simulink model "lb552_usrp_tx_am_fdm"  (R2018b)
settings: Solver=VariableStepAuto  StartTime=0.0  StopTime=inf  RelTol=1e-3
undefined symbols (not defined in the file): fdesignblkfcn, gcbh
libraries: dspvision x3, dspfdesign x3, dsparch4 x2, dspsrcs4 x2, dspmlti4 x2, commsdrhw_v2 x1
settings Model: SimulationMode=accelerator  Creator=Григорий Фокин  LastModifiedBy=Григорий Фокин
settings SFSimCC: SimUseLocalCustomCode=off
settings RTWCC: RTWUseLocalCustomCode=off
settings CodeAppCC: StateflowObjectComments=on

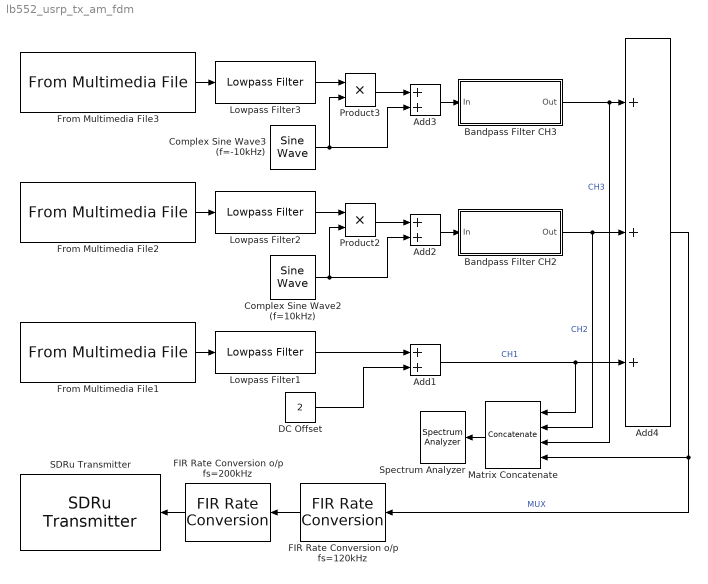
== system lb552_usrp_tx_am_fdm ==
  Add1 : Sum
  Add2 : Sum
  Add3 : Sum
  Add4 : Sum  Inputs=+++
  Bandpass Filter CH2 : Subsystem  DialogController=fdesignblkfcn  InitFcn=fdesignblkfcn(gcbh, {'InitFcn'});  mask(Bandpass Filter){}
      mask help: Design a bandpass filter
      settings: CopyFcn=fdesignblkfcn(gcbh, {'CopyFcn'});
      mask Help: helpview(mapfilelocation('dsp'), 'dspbandpassfilter');
      mask Display: disp('Bandpass');
  Bandpass Filter CH3 : Subsystem  DialogController=fdesignblkfcn  InitFcn=fdesignblkfcn(gcbh, {'InitFcn'});  mask(Bandpass Filter){}
      mask help: Design a bandpass filter
      settings: CopyFcn=fdesignblkfcn(gcbh, {'CopyFcn'});
      mask Help: helpview(mapfilelocation('dsp'), 'dspbandpassfilter');
      mask Display: disp('Bandpass');
  Complex Sine Wave2 (f=10kHz) : dspsrcs4/Sine Wave  Amplitude=2  Frequency=10e3  Phase=0  SampleMode=Discrete  OutComplex=Complex  CompMethod=Trigonometric fcn  TableSize=Speed  SampleTime=1/48e3  SamplesPerFrame=600  ResetState=Restart at time zero  OutputFrames=off  dataType=double  wordLen=16  udDataType=sfix(16)  fracBitsMode=Best precision  numFracBits=15  OutDataTypeStr=double  LastOutDataTypeStr=double
  Complex Sine Wave3 (f=-10kHz) : dspsrcs4/Sine Wave  Amplitude=2  Frequency=-10e3  Phase=0  SampleMode=Discrete  OutComplex=Complex  CompMethod=Trigonometric fcn  TableSize=Speed  SampleTime=1/48e3  SamplesPerFrame=600  ResetState=Restart at time zero  OutputFrames=off  dataType=double  wordLen=16  udDataType=sfix(16)  fracBitsMode=Best precision  numFracBits=15  OutDataTypeStr=double  LastOutDataTypeStr=double
  DC Offset : Constant  Value=2
  FIR Rate Conversion o/p fs=120kHz : dspmlti4/FIR Rate Conversion  FilterSource=Dialog parameters  L=5  h=firpm(100, [0 16000 24000 240e3/2]/(240e3/2), [1 1 0 0], [1 1],20)  M=2  FilterObject=FRC  roundingMode=Floor  overflowMode=off  firstCoeffDataTypeStr=Inherit: Same word length as input  firstCoeffMin=[]  firstCoeffMax=[]  firstCoeffLastDataTypeStr=Inherit: Same word length as input  outputDataTypeStr=Inherit: Same as accumulator  outputMin=[]  outputMax=[]  outputLastDataTypeStr=Inherit: Same as accumulator
      settings: SourceProductName=DSP System Toolbox  SourceProductBaseCode=DS
  FIR Rate Conversion o/p fs=200kHz : dspmlti4/FIR Rate Conversion  FilterSource=Dialog parameters  L=5  h=firpm(100, [0 16e3 24e3 600e3/2]/(600e3/2), [1 1 0 0], [1 1],20)  M=3  FilterObject=FRC  roundingMode=Floor  overflowMode=off  firstCoeffDataTypeStr=Inherit: Same word length as input  firstCoeffMin=[]  firstCoeffMax=[]  firstCoeffLastDataTypeStr=Inherit: Same word length as input  outputDataTypeStr=Inherit: Same as accumulator  outputMin=[]  outputMax=[]  outputLastDataTypeStr=Inherit: Same as accumulator
      settings: SourceProductName=DSP System Toolbox  SourceProductBaseCode=DS
  From Multimedia File1 : dspvision/From Multimedia File  inputFilename=C:\Users\Григорий Фокин\Documents\MATLAB\sut_study\dcsdr\audio_sources\music1_mono48kHz.wav  loop=on  numPlays=inf  outputStreams=Audio only  videoDataType=single  audioDataType=single  inheritSampleTime=on  userDefinedSampleTime=1/30  noAudioOutput=off  isIntensityVideo=off  fourcc=RGB  colorVideoFormat=Separate color signals  outputEOF=off  dataOrg=Column-major  audioFrameSize=600  computeAudioFrameSize=off  outSamplingMode=Sample based
      settings: SourceProductBaseCode=VP
  From Multimedia File2 : dspvision/From Multimedia File  inputFilename=C:\Users\Григорий Фокин\Documents\MATLAB\sut_study\dcsdr\audio_sources\music2_mono48kHz.wav  loop=on  numPlays=inf  outputStreams=Audio only  videoDataType=single  audioDataType=single  inheritSampleTime=on  userDefinedSampleTime=1/30  noAudioOutput=off  isIntensityVideo=off  fourcc=RGB  colorVideoFormat=Separate color signals  outputEOF=off  dataOrg=Column-major  audioFrameSize=600  computeAudioFrameSize=off  outSamplingMode=Sample based
      settings: SourceProductBaseCode=VP
  From Multimedia File3 : dspvision/From Multimedia File  inputFilename=C:\Users\Григорий Фокин\Documents\MATLAB\sut_study\dcsdr\audio_sources\music3_mono48kHz.wav  loop=on  numPlays=inf  outputStreams=Audio only  videoDataType=single  audioDataType=single  inheritSampleTime=on  userDefinedSampleTime=1/30  noAudioOutput=off  isIntensityVideo=off  fourcc=RGB  colorVideoFormat=Separate color signals  outputEOF=off  dataOrg=Column-major  audioFrameSize=600  computeAudioFrameSize=off  outSamplingMode=Sample based
      settings: SourceProductBaseCode=VP
  Lowpass Filter1 : dspfdesign/Lowpass Filter  FilterType=IIR  DesignForMinimumOrder=on  FilterOrder=50  PassbandFrequency=4e3  StopbandFrequency=4.5e3  PassbandRipple=1  StopbandAttenuation=100  InheritSampleRate=off  SampleRate=48e3  SimulateUsing=Interpreted execution  roundingMode=Floor  coeffsDataTypeStr=fixdt(1,16)
  Lowpass Filter2 : dspfdesign/Lowpass Filter  FilterType=IIR  DesignForMinimumOrder=on  FilterOrder=50  PassbandFrequency=4e3  StopbandFrequency=4.5e3  PassbandRipple=1  StopbandAttenuation=100  InheritSampleRate=off  SampleRate=48e3  SimulateUsing=Interpreted execution  roundingMode=Floor  coeffsDataTypeStr=fixdt(1,16)
  Lowpass Filter3 : dspfdesign/Lowpass Filter  FilterType=IIR  DesignForMinimumOrder=on  FilterOrder=50  PassbandFrequency=4e3  StopbandFrequency=4.5e3  PassbandRipple=1  StopbandAttenuation=100  InheritSampleRate=off  SampleRate=48e3  SimulateUsing=Interpreted execution  roundingMode=Floor  coeffsDataTypeStr=fixdt(1,16)
  Matrix Concatenate : Concatenate  NumInputs=4  Mode=Multidimensional array  ConcatenateDimension=2
  Product2 : Product
  Product3 : Product
  SDRu Transmitter : commsdrhw_v2/SDRu Transmitter  rxtx=tx  initializeIPAddress=0  devMap=0  USRP2_IP=192.168.10.2  USRP_IP_X300=192.168.10.2  USRP_IP_X310=192.168.10.2  USRP_serialNumB210=F4E642  platform=B210  prevPlatform=B210  lastIPAddressPopup=192.168.10.2  USRP_ID=F4E642  LastIPAddress=192.168.10.2  ChannelMapping=1  centerFrequencySrc=Dialog  centerFrequency=1200e6  loOffsetSrc=Dialog  loOffset=0  gainSrc=Dialog  gain=70  PPSSource=Internal  clockSource=Internal  masterClkRateParam=6000000  masterClkRateB200=32e6  masterClkRateB210=6e6  masterClkRateX300=200e6  masterClkRateX310=200e6  decimInterpSrc=Dialog  decimInterp=30  USRP2_IP_NUM=[70 52 69 54 52 50]  frameLength=362  TransportDataType=int16  outputDatatype=Same as transport data type  overrunUnderrunPort=off  sampleTime=1  dboardInfo=|  HOST_DATA_PORT=30000  HOST_CONTROL_PORT=30001  USRP2_DATA_PORT=32769  USRP2_CONTROL_PORT=32768  bufferMode=Continuous streaming  EnableBurstMode=off  NumFramesInBurst=100
      | dbid: 0
      |           dbName: 'no db found'
      |          freqMin: 0
      |          freqMax: 0
      |          gainMin: 0
      |          gainMax: 0
      |     gainStepSize: 0
      settings: SourceProductName=Communications System Toolbox Support Package for USRP(R) Radio  SourceProductBaseCode=USRP
  Spectrum Analyzer : SpectrumAnalyzer
  wires:
  From Multimedia File3/1 -> Lowpass Filter3/1
  Lowpass Filter3/1 -> Product3/1
  Complex Sine Wave3 (f=-10kHz)/1 -> Product3/2, Add3/2
  Product3/1 -> Add3/1
  Add3/1 -> Bandpass Filter CH3/1(In)
  From Multimedia File2/1 -> Lowpass Filter2/1
  Lowpass Filter2/1 -> Product2/1
  Complex Sine Wave2 (f=10kHz)/1 -> Add2/2, Product2/2
  Product2/1 -> Add2/1
  Add2/1 -> Bandpass Filter CH2/1(In)
  From Multimedia File1/1 -> Lowpass Filter1/1
  Lowpass Filter1/1 -> Add1/1
  DC Offset/1 -> Add1/2
  Bandpass Filter CH3/1(Out) -> Matrix Concatenate/3, Add4/1  "CH3"
  Bandpass Filter CH2/1(Out) -> Matrix Concatenate/2, Add4/2  "CH2"
  Add1/1 -> Matrix Concatenate/1, Add4/3  "CH1"
  FIR Rate Conversion o/p fs=120kHz/1 -> FIR Rate Conversion o/p fs=200kHz/1
  FIR Rate Conversion o/p fs=200kHz/1 -> SDRu Transmitter/1
  Matrix Concatenate/1 -> Spectrum Analyzer/1
  Add4/1 -> FIR Rate Conversion o/p fs=120kHz/1, Matrix Concatenate/4  "MUX"

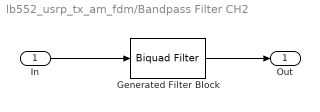
== system lb552_usrp_tx_am_fdm/Bandpass Filter CH2 ==
  In : Inport
  Generated Filter Block : dsparch4/Biquad Filter  Tag=BlockMethodSubSystem  FilterSource=Dialog parameters  CoeffSource=Specify via dialog  FilterObject=BQF  IIRFiltStruct=Direct form II  BiQuadCoeffs=[0.038316192503796788 0 -0.038316192503796788 1 -1.4647964271306377 0.94471193100608075;0.079066094669843379 0 -0.079066094669843379 1 -1.4478872277903894 0.92340777287438669;1.4987829140143871 0 -1.4987829140143871 1 -1.3806603018180272 0.84224281947975999;1.4262911444791184 0 -1.4262911444791184 1 0.58822635838518211 0.83492615482033494;0.12651868683152681 0 -0.12651868683152681 1 0.55132638249904897 0.75583004259253672;0.16278534730934865 0 -0.16278534730934865 1 -1.296689747244494 0.74843901978838578;0.17165110687366125 0 -0.17165110687366125 1 -1.2286258519522211 0.67826050546120453;1.2698273089041143 0 -1.2698273089041143 1 -1.2113783161788545 0.66128071032184788;0.20679428223229829 0 -0.20679428223229829 1 0.4575548300258192 0.59529881813215724;0.24203724548995642 0 -0.24203724548995642 1 -1.1410250658492758 0.59529322698110076;0.25085765032621515 0 -0.25085765032621515 1 -1.0676878443588245 0.53197037847147421;1.1262797117495502 0 -1.1262797117495502 1 -1.0487453100276105 0.51650173917589015;0.28689353541085916 0 -0.28689353541085916 1 0.3519417533947492 0.46218165129526773;0.32503837865502017 0 -0.32503837865502017 1 -0.96986311471358411 0.45593385510682483;1.0469924746795094 0 -1.0469924746795094 1 -0.88468241094327438 0.39740220475460397;0.36600529716476427 0 -0.36600529716476427 1 0.28503939659387562 0.39655389906045346;0.97025355161809479 0 -0.97025355161809479 1 -0.79108046931960629 0.34121276752547192;0.41170205075459598 0 -0.41170205075459598 1 0.21209573444104962 0.3380538505151206;0.89433754435568313 0 -0.89433754435568313 1 -0.68658006847610931 0.2885056716671846;0.81944502214295323 0 -0.81944502214295323 1 0.13161626710115215 0.28686560436176467;0.4635643277972038 0 -0.4635643277972038 1 0.041622402952489035 0.2438446895809836;0.74310982737617481 0 -0.74310982737617481 1 -0.56911862362598775 0.24200449865234008;0.52401642408429749 0 -0.52401642408429749 1 -0.060257140448974483 0.21085064512665316;0.6663474706877075 0 -0.6663474706877075 1 -0.439506581423658 0.20676604963866127;0.59171836614561801 0 -0.59171836614561801 1 -0.17601055769180582 0.1911208065583376;0.62712191993186295 0 -0.62712191993186295 1 -0.30478008617749719 0.18891158557670057;0.69966742183885922 0 -0.69966742183885922 1 -0.23904135382384317 0.18757452699095306;0.55330559254524614 0 -0.55330559254524614 1 -0.11634228576068456 0.19906897851393124;0.76917074247525774 0 -0.76917074247525774 1 -0.37209094308052626 0.19536146214396241;0.48617499002437708 0 -0.48617499002437708 1 -0.0076804609149881825 0.22592720694312463;0.83504112081969528 0 -0.83504112081969528 1 -0.50556036680048511 0.22257689527031324;0.42757746379429307 0 -0.42757746379429307 1 0.087951306871739937 0.26424643599944636;0.37860716298259545 0 -0.37860716298259545 1 -0.62953035756411801 0.2642209496329555;0.85794319827651577 0 -0.85794319827651577 1 -0.74034910133001519 0.31430206283391671;0.3156782373193644 0 -0.3156782373193644 1 0.17290986841503653 0.31151116853219307;0.72504748895787396 0 -0.72504748895787396 1 -0.83908419359333897 0.36896989749244613;0.68432655624176897 0 -0.68432655624176897 1 0.24940543484309963 0.36641429161510974;0.31152694401361014 0 -0.31152694401361014 1 0.31916944212687137 0.42846811137787677;0.68648839199988387 0 -0.68648839199988387 1 -0.92818196779966999 0.42640778321597184;0.30752809817970622 0 -0.30752809817970622 1 0.38347969139959992 0.49774535746443088;0.27169501816632724 0 -0.27169501816632724 1 -1.0099766818316462 0.48596263367743714;0.77277817453089304 0 -0.77277817453089304 1 -1.1048021701758253 0.56332975000387475;0.73508031520027628 0 -0.73508031520027628 1 0.42869230070154496 0.55473049811770636;0.29418562251053465 0 -0.29418562251053465 1 0.48546564941124593 0.6380818919747604;0.23621087503198085 0 -0.23621087503198085 1 -1.1765054758560753 0.62792026806225043;0.92057985047504121 0 -0.92057985047504121 1 -1.26281575076854 0.71287380301019321;0.19821400336650982 0 -0.19821400336650982 1 0.52563846635605715 0.70676158328244532 ...(+4917 chars)]  ScaleValues=[0.036348121033666324;1;1;1;1;1;1;1;1;1;1;1;1;1;1;1;1;1;1;1;1;1;1;1;1;1;1;1;1;1;1;1;1;1;1;1;1;1;1;1;1;1;1;1;1;1;1;1;1;1;1;1;1;1;1;1;1;1;1;1;1;1;1;1;1;1;1;1;1;1;1;1;1;1;1;1;1;1;1;1;1;1;1;1;1;1;1;1;1;1;1;1;1;1;1;1;1;1;1;1;1;1;1;1;1;1]  IC=0  ICnum=0  ICden=0  a0Flag=Warning  optimizeScaleValues=off  ScaleValueMode=Specify via input port (g)  InputProcessing=Columns as channels (frame based)  roundingMode=Floor  overflowMode=off  scaleValueFracLength=14  denProdOutputFracLength=30  denAccumFracLength=30  secondMemoryFracLength=15
      settings: SourceProductName=DSP System Toolbox
  Out : Outport
  wires:
  Generated Filter Block/1 -> Out/1
  In/1 -> Generated Filter Block/1

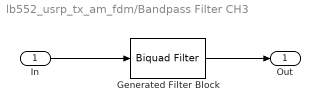
== system lb552_usrp_tx_am_fdm/Bandpass Filter CH3 ==
  In : Inport
  Generated Filter Block : dsparch4/Biquad Filter  Tag=BlockMethodSubSystem  FilterSource=Dialog parameters  CoeffSource=Specify via dialog  FilterObject=BQF  IIRFiltStruct=Direct form II  BiQuadCoeffs=[0.038316192503796788 0 -0.038316192503796788 1 -1.4647964271306377 0.94471193100608075;0.079066094669843379 0 -0.079066094669843379 1 -1.4478872277903894 0.92340777287438669;1.4987829140143871 0 -1.4987829140143871 1 -1.3806603018180272 0.84224281947975999;1.4262911444791184 0 -1.4262911444791184 1 0.58822635838518211 0.83492615482033494;0.12651868683152681 0 -0.12651868683152681 1 0.55132638249904897 0.75583004259253672;0.16278534730934865 0 -0.16278534730934865 1 -1.296689747244494 0.74843901978838578;0.17165110687366125 0 -0.17165110687366125 1 -1.2286258519522211 0.67826050546120453;1.2698273089041143 0 -1.2698273089041143 1 -1.2113783161788545 0.66128071032184788;0.20679428223229829 0 -0.20679428223229829 1 0.4575548300258192 0.59529881813215724;0.24203724548995642 0 -0.24203724548995642 1 -1.1410250658492758 0.59529322698110076;0.25085765032621515 0 -0.25085765032621515 1 -1.0676878443588245 0.53197037847147421;1.1262797117495502 0 -1.1262797117495502 1 -1.0487453100276105 0.51650173917589015;0.28689353541085916 0 -0.28689353541085916 1 0.3519417533947492 0.46218165129526773;0.32503837865502017 0 -0.32503837865502017 1 -0.96986311471358411 0.45593385510682483;1.0469924746795094 0 -1.0469924746795094 1 -0.88468241094327438 0.39740220475460397;0.36600529716476427 0 -0.36600529716476427 1 0.28503939659387562 0.39655389906045346;0.97025355161809479 0 -0.97025355161809479 1 -0.79108046931960629 0.34121276752547192;0.41170205075459598 0 -0.41170205075459598 1 0.21209573444104962 0.3380538505151206;0.89433754435568313 0 -0.89433754435568313 1 -0.68658006847610931 0.2885056716671846;0.81944502214295323 0 -0.81944502214295323 1 0.13161626710115215 0.28686560436176467;0.4635643277972038 0 -0.4635643277972038 1 0.041622402952489035 0.2438446895809836;0.74310982737617481 0 -0.74310982737617481 1 -0.56911862362598775 0.24200449865234008;0.52401642408429749 0 -0.52401642408429749 1 -0.060257140448974483 0.21085064512665316;0.6663474706877075 0 -0.6663474706877075 1 -0.439506581423658 0.20676604963866127;0.59171836614561801 0 -0.59171836614561801 1 -0.17601055769180582 0.1911208065583376;0.62712191993186295 0 -0.62712191993186295 1 -0.30478008617749719 0.18891158557670057;0.69966742183885922 0 -0.69966742183885922 1 -0.23904135382384317 0.18757452699095306;0.55330559254524614 0 -0.55330559254524614 1 -0.11634228576068456 0.19906897851393124;0.76917074247525774 0 -0.76917074247525774 1 -0.37209094308052626 0.19536146214396241;0.48617499002437708 0 -0.48617499002437708 1 -0.0076804609149881825 0.22592720694312463;0.83504112081969528 0 -0.83504112081969528 1 -0.50556036680048511 0.22257689527031324;0.42757746379429307 0 -0.42757746379429307 1 0.087951306871739937 0.26424643599944636;0.37860716298259545 0 -0.37860716298259545 1 -0.62953035756411801 0.2642209496329555;0.85794319827651577 0 -0.85794319827651577 1 -0.74034910133001519 0.31430206283391671;0.3156782373193644 0 -0.3156782373193644 1 0.17290986841503653 0.31151116853219307;0.72504748895787396 0 -0.72504748895787396 1 -0.83908419359333897 0.36896989749244613;0.68432655624176897 0 -0.68432655624176897 1 0.24940543484309963 0.36641429161510974;0.31152694401361014 0 -0.31152694401361014 1 0.31916944212687137 0.42846811137787677;0.68648839199988387 0 -0.68648839199988387 1 -0.92818196779966999 0.42640778321597184;0.30752809817970622 0 -0.30752809817970622 1 0.38347969139959992 0.49774535746443088;0.27169501816632724 0 -0.27169501816632724 1 -1.0099766818316462 0.48596263367743714;0.77277817453089304 0 -0.77277817453089304 1 -1.1048021701758253 0.56332975000387475;0.73508031520027628 0 -0.73508031520027628 1 0.42869230070154496 0.55473049811770636;0.29418562251053465 0 -0.29418562251053465 1 0.48546564941124593 0.6380818919747604;0.23621087503198085 0 -0.23621087503198085 1 -1.1765054758560753 0.62792026806225043;0.92057985047504121 0 -0.92057985047504121 1 -1.26281575076854 0.71287380301019321;0.19821400336650982 0 -0.19821400336650982 1 0.52563846635605715 0.70676158328244532 ...(+4917 chars)]  ScaleValues=[0.036348121033666324;1;1;1;1;1;1;1;1;1;1;1;1;1;1;1;1;1;1;1;1;1;1;1;1;1;1;1;1;1;1;1;1;1;1;1;1;1;1;1;1;1;1;1;1;1;1;1;1;1;1;1;1;1;1;1;1;1;1;1;1;1;1;1;1;1;1;1;1;1;1;1;1;1;1;1;1;1;1;1;1;1;1;1;1;1;1;1;1;1;1;1;1;1;1;1;1;1;1;1;1;1;1;1;1;1]  IC=0  ICnum=0  ICden=0  a0Flag=Warning  optimizeScaleValues=off  ScaleValueMode=Specify via input port (g)  InputProcessing=Columns as channels (frame based)  roundingMode=Floor  overflowMode=off  scaleValueFracLength=14  denProdOutputFracLength=30  denAccumFracLength=30  secondMemoryFracLength=15
      settings: SourceProductName=DSP System Toolbox
  Out : Outport
  wires:
  In/1 -> Generated Filter Block/1
  Generated Filter Block/1 -> Out/1
